simulink model "Grid_modelling_Thermal_V7_ALfix_sheddable"  (R2026a)
settings: Solver=ode45  StopTime=5000  MaxStep=0.01
libraries: sl_discontinuities x10, slpidlib x10, simulink x10
(part 3 of 3)

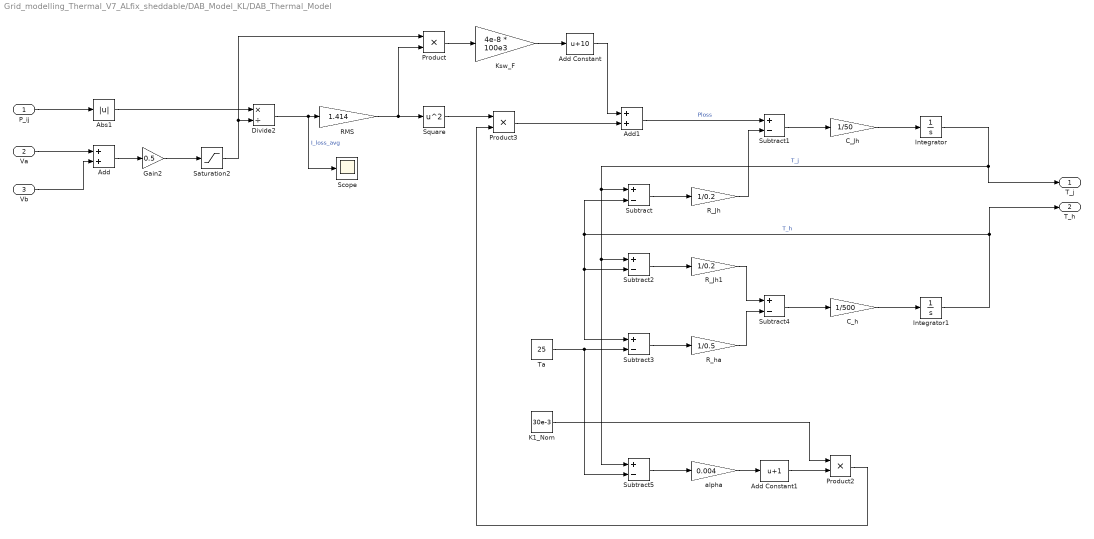
== system Grid_modelling_Thermal_V7_ALfix_sheddable/DAB_Model_KL/DAB_Thermal_Model ==
  P_ij : Inport
  Va : Inport  Port=2
  Vb : Inport  Port=3
  Abs1 : Abs  SaturateOnIntegerOverflow=off
  Add : Sum
  Add Constant : Bias  Bias=10  SaturateOnIntegerOverflow=off
  Add Constant1 : Bias  Bias=1  SaturateOnIntegerOverflow=off
  Add1 : Sum
  C_Jh : Gain  Gain=1/50
  C_h : Gain  Gain=1/500
  Divide2 : Product  Inputs=*/
  Gain2 : Gain  Gain=0.5
  Integrator : Integrator  InitialCondition=25
  Integrator1 : Integrator  InitialCondition=25
  K1_Nom : Constant  Value=30e-3
  Ksw_F : Gain  Gain=4e-8 * 100e3
  Product : Product
  Product2 : Product
  Product3 : Product
  RMS : Gain  Gain=1.414
  R_Jh : Gain  Gain=1/0.2
  R_Jh1 : Gain  Gain=1/0.2
  R_ha : Gain  Gain=1/0.5
  Saturation2 : Saturate  UpperLimit=inf  LowerLimit=1e-3
  Scope : Scope
      settings: ActiveDisplayYMinimum=-2.45667  ActiveDisplayYMaximum=22.11007
  Square : Math  Operator=square
  Subtract{,1..5} (6 alike) : Sum  Inputs=+-
  Ta : Constant  Value=25
  alpha : Gain  Gain=0.004
  T_j : Outport
  T_h : Outport  Port=2
  wires:
  Integrator/1 -> T_j/1, Subtract5/1, Subtract2/1, Subtract/1  "T_j"
  Add1/1 -> Subtract1/1  "Ploss"
  R_ha/1 -> Subtract4/2
  Gain2/1 -> Saturation2/1
  Va/1 -> Add/1
  Integrator1/1 -> T_h/1, Subtract/2, Subtract3/1, Subtract2/2  "T_h"
  R_Jh/1 -> Subtract1/2
  Add/1 -> Gain2/1
  Subtract5/1 -> alpha/1
  Subtract1/1 -> C_Jh/1
  C_h/1 -> Integrator1/1
  Divide2/1 -> Scope/1, RMS/1  "I_loss_avg"
  Product3/1 -> Add1/2
  P_ij/1 -> Abs1/1
  Subtract2/1 -> R_Jh1/1
  alpha/1 -> Add Constant1/1
  Product2/1 -> Product3/2
  C_Jh/1 -> Integrator/1
  Ta/1 -> Subtract5/2, Subtract3/2
  Saturation2/1 -> Product/1, Divide2/2
  R_Jh1/1 -> Subtract4/1
  Subtract/1 -> R_Jh/1
  Abs1/1 -> Divide2/1
  Subtract4/1 -> C_h/1
  Subtract3/1 -> R_ha/1
  Add Constant1/1 -> Product2/2
  Vb/1 -> Add/2
  K1_Nom/1 -> Product2/1
  Square/1 -> Product3/1
  RMS/1 -> Product/2, Square/1
  Product/1 -> Ksw_F/1
  Ksw_F/1 -> Add Constant/1
  Add Constant/1 -> Add1/1

== system Grid_modelling_Thermal_V7_ALfix_sheddable/DAB_Model_KL/thermal_derater ==
  Tj : Inport
  Gain : Gain  Gain=-1
  Gain2 : Gain  Gain=100e3
  If : If  IfExpression=u1 < 125  ElseIfExpressions=u1 > 125 & u1 < 175, u1 > 175  ShowElse=off
  If Action Subsystem : Subsystem  TreatAsAtomicUnit=on
  If Action Subsystem1 : Subsystem  TreatAsAtomicUnit=on
  If Action Subsystem2 : Subsystem  TreatAsAtomicUnit=on
  Merge : Merge  Inputs=3
  Saturation2 : Saturate  UpperLimit=1  LowerLimit=0
  Scope : Scope
      settings: ActiveDisplayYMinimum=0.9  ActiveDisplayYMaximum=1.1  DataLoggingVariableName=ScopeData2
  derate_pos : Outport
  derate_neg : Outport  Port=2
  wires:
  If/1 -> If Action Subsystem/Action
  Tj/1 -> If/1, If Action Subsystem1/1(Tj)
  If/3 -> If Action Subsystem2/Action
  If/2 -> If Action Subsystem1/Action
  If Action Subsystem2/1(Out1) -> Merge/3
  If Action Subsystem1/1(Out1) -> Merge/2
  Merge/1 -> Saturation2/1
  If Action Subsystem/1(Out1) -> Merge/1
  Gain2/1 -> derate_pos/1, Gain/1
  Saturation2/1 -> Scope/1, Gain2/1  "DAB_KL_derate_factor"
  Gain/1 -> derate_neg/1

== system Grid_modelling_Thermal_V7_ALfix_sheddable/source_bus_model_A/Bus_Bar_Thermal_Model ==
  i_src_k : Inport
  Add Constant : Bias  Bias=1  SaturateOnIntegerOverflow=off
  Add1 : Sum
  Constant2 : Constant  Value=25
  Cth_bus : Gain  Gain=1 / 2000
  Integrator1 : Integrator  InitialCondition=25
  Product1 : Product
  Product2 : Product
  R_bus_nom : Constant  Value=0.5e-3
  R_contact : Constant  Value=50e-6
  Rth_bus : Gain  Gain=1/0.6
  Square : Math  Operator=square
  Subtract1 : Sum  Inputs=+-
  Subtract2 : Sum  Inputs=+-
  alpha_copper : Gain  Gain=0.00403
  no_of_contacts : Gain  Gain=10
  T_bus : Outport
  wires:
  Constant2/1 -> Subtract1/2
  Add Constant/1 -> Product2/1
  Product2/1 -> Add1/1
  Cth_bus/1 -> Integrator1/1
  Integrator1/1 -> T_bus/1, Subtract1/1  "T_bus"
  Subtract2/1 -> Cth_bus/1
  alpha_copper/1 -> Add Constant/1
  Subtract1/1 -> alpha_copper/1, Rth_bus/1
  Square/1 -> Product1/1
  Rth_bus/1 -> Subtract2/2
  R_contact/1 -> no_of_contacts/1
  Add1/1 -> Product1/2
  no_of_contacts/1 -> Add1/2
  Product1/1 -> Subtract2/1
  R_bus_nom/1 -> Product2/2
  i_src_k/1 -> Square/1

== system Grid_modelling_Thermal_V7_ALfix_sheddable/source_bus_model_B/Bus_Bar_Thermal_Model ==
  i_src_k : Inport
  Add Constant : Bias  Bias=1  SaturateOnIntegerOverflow=off
  Add1 : Sum
  Constant2 : Constant  Value=25
  Cth_bus : Gain  Gain=1 / 2000
  Integrator1 : Integrator  InitialCondition=25
  Product1 : Product
  Product2 : Product
  R_bus_nom : Constant  Value=0.5e-3
  R_contact : Constant  Value=50e-6
  Rth_bus : Gain  Gain=1/0.6
  Square : Math  Operator=square
  Subtract1 : Sum  Inputs=+-
  Subtract2 : Sum  Inputs=+-
  alpha_copper : Gain  Gain=0.00403
  no_of_contacts : Gain  Gain=10
  T_bus : Outport
  wires:
  Constant2/1 -> Subtract1/2
  Add Constant/1 -> Product2/1
  Product2/1 -> Add1/1
  Cth_bus/1 -> Integrator1/1
  Integrator1/1 -> T_bus/1, Subtract1/1  "T_bus"
  Subtract2/1 -> Cth_bus/1
  alpha_copper/1 -> Add Constant/1
  Subtract1/1 -> alpha_copper/1, Rth_bus/1
  Square/1 -> Product1/1
  Rth_bus/1 -> Subtract2/2
  R_contact/1 -> no_of_contacts/1
  Add1/1 -> Product1/2
  no_of_contacts/1 -> Add1/2
  Product1/1 -> Subtract2/1
  R_bus_nom/1 -> Product2/2
  i_src_k/1 -> Square/1

== system Grid_modelling_Thermal_V7_ALfix_sheddable/source_bus_model_C/Bus_Bar_Thermal_Model ==
  i_src_k : Inport
  Add Constant : Bias  Bias=1  SaturateOnIntegerOverflow=off
  Add1 : Sum
  Constant2 : Constant  Value=25
  Cth_bus : Gain  Gain=1 / 2000
  Integrator1 : Integrator  InitialCondition=25
  Product1 : Product
  Product2 : Product
  R_bus_nom : Constant  Value=0.5e-3
  R_contact : Constant  Value=50e-6
  Rth_bus : Gain  Gain=1/0.6
  Square : Math  Operator=square
  Subtract1 : Sum  Inputs=+-
  Subtract2 : Sum  Inputs=+-
  alpha_copper : Gain  Gain=0.00403
  no_of_contacts : Gain  Gain=10
  T_bus : Outport
  wires:
  Constant2/1 -> Subtract1/2
  Add Constant/1 -> Product2/1
  Product2/1 -> Add1/1
  Cth_bus/1 -> Integrator1/1
  Integrator1/1 -> T_bus/1, Subtract1/1  "T_bus"
  Subtract2/1 -> Cth_bus/1
  alpha_copper/1 -> Add Constant/1
  Subtract1/1 -> alpha_copper/1, Rth_bus/1
  Square/1 -> Product1/1
  Rth_bus/1 -> Subtract2/2
  R_contact/1 -> no_of_contacts/1
  Add1/1 -> Product1/2
  no_of_contacts/1 -> Add1/2
  Product1/1 -> Subtract2/1
  R_bus_nom/1 -> Product2/2
  i_src_k/1 -> Square/1

== system Grid_modelling_Thermal_V7_ALfix_sheddable/source_bus_model_D/Bus_Bar_Thermal_Model ==
  i_src_k : Inport
  Add Constant : Bias  Bias=1  SaturateOnIntegerOverflow=off
  Add1 : Sum
  Constant2 : Constant  Value=25
  Cth_bus : Gain  Gain=1 / 2000
  Integrator1 : Integrator  InitialCondition=25
  Product1 : Product
  Product2 : Product
  R_bus_nom : Constant  Value=0.5e-3
  R_contact : Constant  Value=50e-6
  Rth_bus : Gain  Gain=1/0.6
  Square : Math  Operator=square
  Subtract1 : Sum  Inputs=+-
  Subtract2 : Sum  Inputs=+-
  alpha_copper : Gain  Gain=0.00403
  no_of_contacts : Gain  Gain=10
  T_bus : Outport
  wires:
  Constant2/1 -> Subtract1/2
  Add Constant/1 -> Product2/1
  Product2/1 -> Add1/1
  Cth_bus/1 -> Integrator1/1
  Integrator1/1 -> T_bus/1, Subtract1/1  "T_bus"
  Subtract2/1 -> Cth_bus/1
  alpha_copper/1 -> Add Constant/1
  Subtract1/1 -> alpha_copper/1, Rth_bus/1
  Square/1 -> Product1/1
  Rth_bus/1 -> Subtract2/2
  R_contact/1 -> no_of_contacts/1
  Add1/1 -> Product1/2
  no_of_contacts/1 -> Add1/2
  Product1/1 -> Subtract2/1
  R_bus_nom/1 -> Product2/2
  i_src_k/1 -> Square/1

== system Grid_modelling_Thermal_V7_ALfix_sheddable/source_bus_model_E/Bus_Bar_Thermal_Model ==
  i_src_k : Inport
  Add Constant : Bias  Bias=1  SaturateOnIntegerOverflow=off
  Add1 : Sum
  Constant2 : Constant  Value=25
  Cth_bus : Gain  Gain=1 / 2000
  Integrator1 : Integrator  InitialCondition=25
  Product1 : Product
  Product2 : Product
  R_bus_nom : Constant  Value=0.5e-3
  R_contact : Constant  Value=50e-6
  Rth_bus : Gain  Gain=1/0.6
  Square : Math  Operator=square
  Subtract1 : Sum  Inputs=+-
  Subtract2 : Sum  Inputs=+-
  alpha_copper : Gain  Gain=0.00403
  no_of_contacts : Gain  Gain=10
  T_bus : Outport
  wires:
  Constant2/1 -> Subtract1/2
  Add Constant/1 -> Product2/1
  Product2/1 -> Add1/1
  Cth_bus/1 -> Integrator1/1
  Integrator1/1 -> T_bus/1, Subtract1/1  "T_bus"
  Subtract2/1 -> Cth_bus/1
  alpha_copper/1 -> Add Constant/1
  Subtract1/1 -> alpha_copper/1, Rth_bus/1
  Square/1 -> Product1/1
  Rth_bus/1 -> Subtract2/2
  R_contact/1 -> no_of_contacts/1
  Add1/1 -> Product1/2
  no_of_contacts/1 -> Add1/2
  Product1/1 -> Subtract2/1
  R_bus_nom/1 -> Product2/2
  i_src_k/1 -> Square/1

== system Grid_modelling_Thermal_V7_ALfix_sheddable/source_bus_model_F/Bus_Bar_Thermal_Model ==
  i_src_k : Inport
  Add Constant : Bias  Bias=1  SaturateOnIntegerOverflow=off
  Add1 : Sum
  Constant2 : Constant  Value=25
  Cth_bus : Gain  Gain=1 / 2000
  Integrator1 : Integrator  InitialCondition=25
  Product1 : Product
  Product2 : Product
  R_bus_nom : Constant  Value=0.5e-3
  R_contact : Constant  Value=50e-6
  Rth_bus : Gain  Gain=1/0.6
  Square : Math  Operator=square
  Subtract1 : Sum  Inputs=+-
  Subtract2 : Sum  Inputs=+-
  alpha_copper : Gain  Gain=0.00403
  no_of_contacts : Gain  Gain=10
  T_bus : Outport
  wires:
  Constant2/1 -> Subtract1/2
  Add Constant/1 -> Product2/1
  Product2/1 -> Add1/1
  Cth_bus/1 -> Integrator1/1
  Integrator1/1 -> T_bus/1, Subtract1/1  "T_bus"
  Subtract2/1 -> Cth_bus/1
  alpha_copper/1 -> Add Constant/1
  Subtract1/1 -> alpha_copper/1, Rth_bus/1
  Square/1 -> Product1/1
  Rth_bus/1 -> Subtract2/2
  R_contact/1 -> no_of_contacts/1
  Add1/1 -> Product1/2
  no_of_contacts/1 -> Add1/2
  Product1/1 -> Subtract2/1
  R_bus_nom/1 -> Product2/2
  i_src_k/1 -> Square/1

== system Grid_modelling_Thermal_V7_ALfix_sheddable/source_bus_model_G/Bus_Bar_Thermal_Model ==
  i_src_k : Inport
  Add Constant : Bias  Bias=1  SaturateOnIntegerOverflow=off
  Add1 : Sum
  Constant2 : Constant  Value=25
  Cth_bus : Gain  Gain=1 / 2000
  Integrator1 : Integrator  InitialCondition=25
  Product1 : Product
  Product2 : Product
  R_bus_nom : Constant  Value=0.5e-3
  R_contact : Constant  Value=50e-6
  Rth_bus : Gain  Gain=1/0.6
  Square : Math  Operator=square
  Subtract1 : Sum  Inputs=+-
  Subtract2 : Sum  Inputs=+-
  alpha_copper : Gain  Gain=0.00403
  no_of_contacts : Gain  Gain=10
  T_bus : Outport
  wires:
  Constant2/1 -> Subtract1/2
  Add Constant/1 -> Product2/1
  Product2/1 -> Add1/1
  Cth_bus/1 -> Integrator1/1
  Integrator1/1 -> T_bus/1, Subtract1/1  "T_bus"
  Subtract2/1 -> Cth_bus/1
  alpha_copper/1 -> Add Constant/1
  Subtract1/1 -> alpha_copper/1, Rth_bus/1
  Square/1 -> Product1/1
  Rth_bus/1 -> Subtract2/2
  R_contact/1 -> no_of_contacts/1
  Add1/1 -> Product1/2
  no_of_contacts/1 -> Add1/2
  Product1/1 -> Subtract2/1
  R_bus_nom/1 -> Product2/2
  i_src_k/1 -> Square/1

== system Grid_modelling_Thermal_V7_ALfix_sheddable/source_bus_model_H/Bus_Bar_Thermal_Model ==
  i_src_k : Inport
  Add Constant : Bias  Bias=1  SaturateOnIntegerOverflow=off
  Add1 : Sum
  Constant2 : Constant  Value=25
  Cth_bus : Gain  Gain=1 / 2000
  Integrator1 : Integrator  InitialCondition=25
  Product1 : Product
  Product2 : Product
  R_bus_nom : Constant  Value=0.5e-3
  R_contact : Constant  Value=50e-6
  Rth_bus : Gain  Gain=1/0.6
  Square : Math  Operator=square
  Subtract1 : Sum  Inputs=+-
  Subtract2 : Sum  Inputs=+-
  alpha_copper : Gain  Gain=0.00403
  no_of_contacts : Gain  Gain=10
  T_bus : Outport
  wires:
  Constant2/1 -> Subtract1/2
  Add Constant/1 -> Product2/1
  Product2/1 -> Add1/1
  Cth_bus/1 -> Integrator1/1
  Integrator1/1 -> T_bus/1, Subtract1/1  "T_bus"
  Subtract2/1 -> Cth_bus/1
  alpha_copper/1 -> Add Constant/1
  Subtract1/1 -> alpha_copper/1, Rth_bus/1
  Square/1 -> Product1/1
  Rth_bus/1 -> Subtract2/2
  R_contact/1 -> no_of_contacts/1
  Add1/1 -> Product1/2
  no_of_contacts/1 -> Add1/2
  Product1/1 -> Subtract2/1
  R_bus_nom/1 -> Product2/2
  i_src_k/1 -> Square/1

== system Grid_modelling_Thermal_V7_ALfix_sheddable/source_bus_model_K/Bus_Bar_Thermal_Model ==
  i_src_k : Inport
  Add Constant : Bias  Bias=1  SaturateOnIntegerOverflow=off
  Add1 : Sum
  Constant2 : Constant  Value=25
  Cth_bus : Gain  Gain=1 / 2000
  Integrator1 : Integrator  InitialCondition=25
  Product1 : Product
  Product2 : Product
  R_bus_nom : Constant  Value=0.5e-3
  R_contact : Constant  Value=50e-6
  Rth_bus : Gain  Gain=1/0.6
  Square : Math  Operator=square
  Subtract1 : Sum  Inputs=+-
  Subtract2 : Sum  Inputs=+-
  alpha_copper : Gain  Gain=0.00403
  no_of_contacts : Gain  Gain=10
  T_bus : Outport
  wires:
  Constant2/1 -> Subtract1/2
  Add Constant/1 -> Product2/1
  Product2/1 -> Add1/1
  Cth_bus/1 -> Integrator1/1
  Integrator1/1 -> T_bus/1, Subtract1/1  "T_bus"
  Subtract2/1 -> Cth_bus/1
  alpha_copper/1 -> Add Constant/1
  Subtract1/1 -> alpha_copper/1, Rth_bus/1
  Square/1 -> Product1/1
  Rth_bus/1 -> Subtract2/2
  R_contact/1 -> no_of_contacts/1
  Add1/1 -> Product1/2
  no_of_contacts/1 -> Add1/2
  Product1/1 -> Subtract2/1
  R_bus_nom/1 -> Product2/2
  i_src_k/1 -> Square/1

== system Grid_modelling_Thermal_V7_ALfix_sheddable/source_bus_model_L/Bus_Bar_Thermal_Model ==
  i_src_k : Inport
  Add Constant : Bias  Bias=1  SaturateOnIntegerOverflow=off
  Add1 : Sum
  Constant2 : Constant  Value=25
  Cth_bus : Gain  Gain=1 / 2000
  Integrator1 : Integrator  InitialCondition=25
  Product1 : Product
  Product2 : Product
  R_bus_nom : Constant  Value=0.5e-3
  R_contact : Constant  Value=50e-6
  Rth_bus : Gain  Gain=1/0.6
  Square : Math  Operator=square
  Subtract1 : Sum  Inputs=+-
  Subtract2 : Sum  Inputs=+-
  alpha_copper : Gain  Gain=0.00403
  no_of_contacts : Gain  Gain=10
  T_bus : Outport
  wires:
  Constant2/1 -> Subtract1/2
  Add Constant/1 -> Product2/1
  Product2/1 -> Add1/1
  Cth_bus/1 -> Integrator1/1
  Integrator1/1 -> T_bus/1, Subtract1/1  "T_bus"
  Subtract2/1 -> Cth_bus/1
  alpha_copper/1 -> Add Constant/1
  Subtract1/1 -> alpha_copper/1, Rth_bus/1
  Square/1 -> Product1/1
  Rth_bus/1 -> Subtract2/2
  R_contact/1 -> no_of_contacts/1
  Add1/1 -> Product1/2
  no_of_contacts/1 -> Add1/2
  Product1/1 -> Subtract2/1
  R_bus_nom/1 -> Product2/2
  i_src_k/1 -> Square/1

== system Grid_modelling_Thermal_V7_ALfix_sheddable/DAB_Model_AB/thermal_derater/If Action Subsystem ==
  Action Port : ActionPort  ActionPortLabel=if(u1 < 125)
  Constant : Constant
  Out1 : Outport
  wires:
  Constant/1 -> Out1/1

== system Grid_modelling_Thermal_V7_ALfix_sheddable/DAB_Model_AB/thermal_derater/If Action Subsystem1 ==
  Tj : Inport
  Action Port : ActionPort  ActionPortLabel=elseif(u1 > 125 & u1 < 175)
  Divide : Product  Inputs=*/
  Subtract : Sum  Inputs=+-
  Subtract1 : Sum  Inputs=+-
  Tderate : Constant  Value=125
  Tmax : Constant  Value=175
  Out1 : Outport
  wires:
  Divide/1 -> Out1/1
  Tj/1 -> Subtract/2
  Tmax/1 -> Subtract1/1, Subtract/1
  Tderate/1 -> Subtract1/2
  Subtract/1 -> Divide/1
  Subtract1/1 -> Divide/2

== system Grid_modelling_Thermal_V7_ALfix_sheddable/DAB_Model_AB/thermal_derater/If Action Subsystem2 ==
  Action Port : ActionPort  ActionPortLabel=elseif( u1 > 175)
  Constant : Constant
  Out1 : Outport
  wires:
  Constant/1 -> Out1/1

== system Grid_modelling_Thermal_V7_ALfix_sheddable/DAB_Model_AL/thermal_derater/If Action Subsystem ==
  Action Port : ActionPort  ActionPortLabel=if(u1 < 125)
  Constant : Constant
  Out1 : Outport
  wires:
  Constant/1 -> Out1/1

== system Grid_modelling_Thermal_V7_ALfix_sheddable/DAB_Model_AL/thermal_derater/If Action Subsystem1 ==
  Tj : Inport
  Action Port : ActionPort  ActionPortLabel=elseif(u1 > 125 & u1 < 175)
  Divide : Product  Inputs=*/
  Subtract : Sum  Inputs=+-
  Subtract1 : Sum  Inputs=+-
  Tderate : Constant  Value=125
  Tmax : Constant  Value=175
  Out1 : Outport
  wires:
  Divide/1 -> Out1/1
  Tj/1 -> Subtract/2
  Tmax/1 -> Subtract1/1, Subtract/1
  Tderate/1 -> Subtract1/2
  Subtract/1 -> Divide/1
  Subtract1/1 -> Divide/2

== system Grid_modelling_Thermal_V7_ALfix_sheddable/DAB_Model_AL/thermal_derater/If Action Subsystem2 ==
  Action Port : ActionPort  ActionPortLabel=elseif( u1 > 175)
  Constant : Constant
  Out1 : Outport
  wires:
  Constant/1 -> Out1/1

== system Grid_modelling_Thermal_V7_ALfix_sheddable/DAB_Model_BC/thermal_derater/If Action Subsystem ==
  Action Port : ActionPort  ActionPortLabel=if(u1 < 125)
  Constant : Constant
  Out1 : Outport
  wires:
  Constant/1 -> Out1/1

== system Grid_modelling_Thermal_V7_ALfix_sheddable/DAB_Model_BC/thermal_derater/If Action Subsystem1 ==
  Tj : Inport
  Action Port : ActionPort  ActionPortLabel=elseif(u1 > 125 & u1 < 175)
  Divide : Product  Inputs=*/
  Subtract : Sum  Inputs=+-
  Subtract1 : Sum  Inputs=+-
  Tderate : Constant  Value=125
  Tmax : Constant  Value=175
  Out1 : Outport
  wires:
  Divide/1 -> Out1/1
  Tj/1 -> Subtract/2
  Tmax/1 -> Subtract1/1, Subtract/1
  Tderate/1 -> Subtract1/2
  Subtract/1 -> Divide/1
  Subtract1/1 -> Divide/2

== system Grid_modelling_Thermal_V7_ALfix_sheddable/DAB_Model_BC/thermal_derater/If Action Subsystem2 ==
  Action Port : ActionPort  ActionPortLabel=elseif( u1 > 175)
  Constant : Constant
  Out1 : Outport
  wires:
  Constant/1 -> Out1/1

== system Grid_modelling_Thermal_V7_ALfix_sheddable/DAB_Model_CD/thermal_derater/If Action Subsystem ==
  Action Port : ActionPort  ActionPortLabel=if(u1 < 125)
  Constant : Constant
  Out1 : Outport
  wires:
  Constant/1 -> Out1/1

== system Grid_modelling_Thermal_V7_ALfix_sheddable/DAB_Model_CD/thermal_derater/If Action Subsystem1 ==
  Tj : Inport
  Action Port : ActionPort  ActionPortLabel=elseif(u1 > 125 & u1 < 175)
  Divide : Product  Inputs=*/
  Subtract : Sum  Inputs=+-
  Subtract1 : Sum  Inputs=+-
  Tderate : Constant  Value=125
  Tmax : Constant  Value=175
  Out1 : Outport
  wires:
  Divide/1 -> Out1/1
  Tj/1 -> Subtract/2
  Tmax/1 -> Subtract1/1, Subtract/1
  Tderate/1 -> Subtract1/2
  Subtract/1 -> Divide/1
  Subtract1/1 -> Divide/2

== system Grid_modelling_Thermal_V7_ALfix_sheddable/DAB_Model_CD/thermal_derater/If Action Subsystem2 ==
  Action Port : ActionPort  ActionPortLabel=elseif( u1 > 175)
  Constant : Constant
  Out1 : Outport
  wires:
  Constant/1 -> Out1/1

== system Grid_modelling_Thermal_V7_ALfix_sheddable/DAB_Model_DE/thermal_derater/If Action Subsystem ==
  Action Port : ActionPort  ActionPortLabel=if(u1 < 125)
  Constant : Constant
  Out1 : Outport
  wires:
  Constant/1 -> Out1/1

== system Grid_modelling_Thermal_V7_ALfix_sheddable/DAB_Model_DE/thermal_derater/If Action Subsystem1 ==
  Tj : Inport
  Action Port : ActionPort  ActionPortLabel=elseif(u1 > 125 & u1 < 175)
  Divide : Product  Inputs=*/
  Subtract : Sum  Inputs=+-
  Subtract1 : Sum  Inputs=+-
  Tderate : Constant  Value=125
  Tmax : Constant  Value=175
  Out1 : Outport
  wires:
  Divide/1 -> Out1/1
  Tj/1 -> Subtract/2
  Tmax/1 -> Subtract1/1, Subtract/1
  Tderate/1 -> Subtract1/2
  Subtract/1 -> Divide/1
  Subtract1/1 -> Divide/2

== system Grid_modelling_Thermal_V7_ALfix_sheddable/DAB_Model_DE/thermal_derater/If Action Subsystem2 ==
  Action Port : ActionPort  ActionPortLabel=elseif( u1 > 175)
  Constant : Constant
  Out1 : Outport
  wires:
  Constant/1 -> Out1/1

== system Grid_modelling_Thermal_V7_ALfix_sheddable/DAB_Model_EF/thermal_derater/If Action Subsystem ==
  Action Port : ActionPort  ActionPortLabel=if(u1 < 125)
  Constant : Constant
  Out1 : Outport
  wires:
  Constant/1 -> Out1/1

== system Grid_modelling_Thermal_V7_ALfix_sheddable/DAB_Model_EF/thermal_derater/If Action Subsystem1 ==
  Tj : Inport
  Action Port : ActionPort  ActionPortLabel=elseif(u1 > 125 & u1 < 175)
  Divide : Product  Inputs=*/
  Subtract : Sum  Inputs=+-
  Subtract1 : Sum  Inputs=+-
  Tderate : Constant  Value=125
  Tmax : Constant  Value=175
  Out1 : Outport
  wires:
  Divide/1 -> Out1/1
  Tj/1 -> Subtract/2
  Tmax/1 -> Subtract1/1, Subtract/1
  Tderate/1 -> Subtract1/2
  Subtract/1 -> Divide/1
  Subtract1/1 -> Divide/2

== system Grid_modelling_Thermal_V7_ALfix_sheddable/DAB_Model_EF/thermal_derater/If Action Subsystem2 ==
  Action Port : ActionPort  ActionPortLabel=elseif( u1 > 175)
  Constant : Constant
  Out1 : Outport
  wires:
  Constant/1 -> Out1/1

== system Grid_modelling_Thermal_V7_ALfix_sheddable/DAB_Model_FG/thermal_derater/If Action Subsystem ==
  Action Port : ActionPort  ActionPortLabel=if(u1 < 125)
  Constant : Constant
  Out1 : Outport
  wires:
  Constant/1 -> Out1/1

== system Grid_modelling_Thermal_V7_ALfix_sheddable/DAB_Model_FG/thermal_derater/If Action Subsystem1 ==
  Tj : Inport
  Action Port : ActionPort  ActionPortLabel=elseif(u1 > 125 & u1 < 175)
  Divide : Product  Inputs=*/
  Subtract : Sum  Inputs=+-
  Subtract1 : Sum  Inputs=+-
  Tderate : Constant  Value=125
  Tmax : Constant  Value=175
  Out1 : Outport
  wires:
  Divide/1 -> Out1/1
  Tj/1 -> Subtract/2
  Tmax/1 -> Subtract1/1, Subtract/1
  Tderate/1 -> Subtract1/2
  Subtract/1 -> Divide/1
  Subtract1/1 -> Divide/2

== system Grid_modelling_Thermal_V7_ALfix_sheddable/DAB_Model_FG/thermal_derater/If Action Subsystem2 ==
  Action Port : ActionPort  ActionPortLabel=elseif( u1 > 175)
  Constant : Constant
  Out1 : Outport
  wires:
  Constant/1 -> Out1/1

== system Grid_modelling_Thermal_V7_ALfix_sheddable/DAB_Model_GH/thermal_derater/If Action Subsystem ==
  Action Port : ActionPort  ActionPortLabel=if(u1 < 125)
  Constant : Constant
  Out1 : Outport
  wires:
  Constant/1 -> Out1/1

== system Grid_modelling_Thermal_V7_ALfix_sheddable/DAB_Model_GH/thermal_derater/If Action Subsystem1 ==
  Tj : Inport
  Action Port : ActionPort  ActionPortLabel=elseif(u1 > 125 & u1 < 175)
  Divide : Product  Inputs=*/
  Subtract : Sum  Inputs=+-
  Subtract1 : Sum  Inputs=+-
  Tderate : Constant  Value=125
  Tmax : Constant  Value=175
  Out1 : Outport
  wires:
  Divide/1 -> Out1/1
  Tj/1 -> Subtract/2
  Tmax/1 -> Subtract1/1, Subtract/1
  Tderate/1 -> Subtract1/2
  Subtract/1 -> Divide/1
  Subtract1/1 -> Divide/2

== system Grid_modelling_Thermal_V7_ALfix_sheddable/DAB_Model_GH/thermal_derater/If Action Subsystem2 ==
  Action Port : ActionPort  ActionPortLabel=elseif( u1 > 175)
  Constant : Constant
  Out1 : Outport
  wires:
  Constant/1 -> Out1/1

== system Grid_modelling_Thermal_V7_ALfix_sheddable/DAB_Model_HK/thermal_derater/If Action Subsystem ==
  Action Port : ActionPort  ActionPortLabel=if(u1 < 125)
  Constant : Constant
  Out1 : Outport
  wires:
  Constant/1 -> Out1/1

== system Grid_modelling_Thermal_V7_ALfix_sheddable/DAB_Model_HK/thermal_derater/If Action Subsystem1 ==
  Tj : Inport
  Action Port : ActionPort  ActionPortLabel=elseif(u1 > 125 & u1 < 175)
  Divide : Product  Inputs=*/
  Subtract : Sum  Inputs=+-
  Subtract1 : Sum  Inputs=+-
  Tderate : Constant  Value=125
  Tmax : Constant  Value=175
  Out1 : Outport
  wires:
  Divide/1 -> Out1/1
  Tj/1 -> Subtract/2
  Tmax/1 -> Subtract1/1, Subtract/1
  Tderate/1 -> Subtract1/2
  Subtract/1 -> Divide/1
  Subtract1/1 -> Divide/2

== system Grid_modelling_Thermal_V7_ALfix_sheddable/DAB_Model_HK/thermal_derater/If Action Subsystem2 ==
  Action Port : ActionPort  ActionPortLabel=elseif( u1 > 175)
  Constant : Constant
  Out1 : Outport
  wires:
  Constant/1 -> Out1/1

== system Grid_modelling_Thermal_V7_ALfix_sheddable/DAB_Model_KL/thermal_derater/If Action Subsystem ==
  Action Port : ActionPort  ActionPortLabel=if(u1 < 125)
  Constant : Constant
  Out1 : Outport
  wires:
  Constant/1 -> Out1/1

== system Grid_modelling_Thermal_V7_ALfix_sheddable/DAB_Model_KL/thermal_derater/If Action Subsystem1 ==
  Tj : Inport
  Action Port : ActionPort  ActionPortLabel=elseif(u1 > 125 & u1 < 175)
  Divide : Product  Inputs=*/
  Subtract : Sum  Inputs=+-
  Subtract1 : Sum  Inputs=+-
  Tderate : Constant  Value=125
  Tmax : Constant  Value=175
  Out1 : Outport
  wires:
  Divide/1 -> Out1/1
  Tj/1 -> Subtract/2
  Tmax/1 -> Subtract1/1, Subtract/1
  Tderate/1 -> Subtract1/2
  Subtract/1 -> Divide/1
  Subtract1/1 -> Divide/2

== system Grid_modelling_Thermal_V7_ALfix_sheddable/DAB_Model_KL/thermal_derater/If Action Subsystem2 ==
  Action Port : ActionPort  ActionPortLabel=elseif( u1 > 175)
  Constant : Constant
  Out1 : Outport
  wires:
  Constant/1 -> Out1/1
